simulink model "mBraccioHW"  (R2021a)
settings: Solver=FixedStepAuto  StartTime=0.0  StopTime=inf  RelTol=1e-3  EnableMultiTasking=on
InitFcn:
  | % oJointBase      = classes.Joint(deg2rad(0)-pi/2, deg2rad(180)-pi/2);
  | % oJointShoulder  = classes.Joint(deg2rad(15)-pi/2, deg2rad(165)-pi/2);
  | % oJointElbow     = classes.Joint(deg2rad(0)-pi/2, deg2rad(180)-pi/2);
  | % oJointPitch     = classes.Joint(deg2rad(0)-pi/2, deg2rad(180)-pi/2);
  | % oJointWrist     = classes.Joint(deg2rad(0)-pi/2, deg2rad(180)-pi/2);
  | 
  | % oLinkGround     = classes.Link(70);
  | % oLinkArm        = classes.Link(125);
  | % oLinkForearm    = classes.Link(125);
  | % oLinkHand       = classes.Link(185);
undefined symbols (not defined in the file): adHome, adWS
libraries: arduinolib x13
settings Model: SILPILModeSetting=veronly  ExtModeTrigDuration=2  Creator=angelo  LastModifiedBy=angelo
settings OptimizationCC: EnhancedBackFolding=on  PassReuseOutputArgsAs=Individual arguments  ZeroExternalMemoryAtStartup=off  ZeroInternalMemoryAtStartup=off  MaxStackSize=64  OptimizeBlockOrder=speed  DifferentSizesBufferReuse=on  OptimizationCustomize=off  EfficientTunableParamExpr=on
settings DebuggingCC: ParameterTunabilityLossMsg=error
settings HardwareCC: ProdBitPerInt=16  ProdBitPerPointer=16  ProdBitPerSizeT=16  ProdBitPerPtrDiffT=16  ProdLargestAtomicFloat=None  ProdWordSize=8  ProdHWDeviceType=Atmel->AVR
settings SFSimCC: MATLABDynamicMemAlloc=off
settings RTWCC: SystemTargetFile=ert.tlc  HardwareBoard=Arduino Mega 2560  TemplateMakefile=ert_default_tmf  Toolchain=Arduino AVR  BuildConfiguration=Faster Runs
settings CodeAppCC: ForceParamTrailComments=on  IgnoreCustomStorageClasses=off  OperatorAnnotations=on  SimulinkDataObjDesc=on  SFDataObjDesc=on  InsertBlockDesc=on
settings ERTTargetCC: SupportContinuousTime=on  SupportVariableSizeSignals=on  ExtModeStaticAllocSize=2048

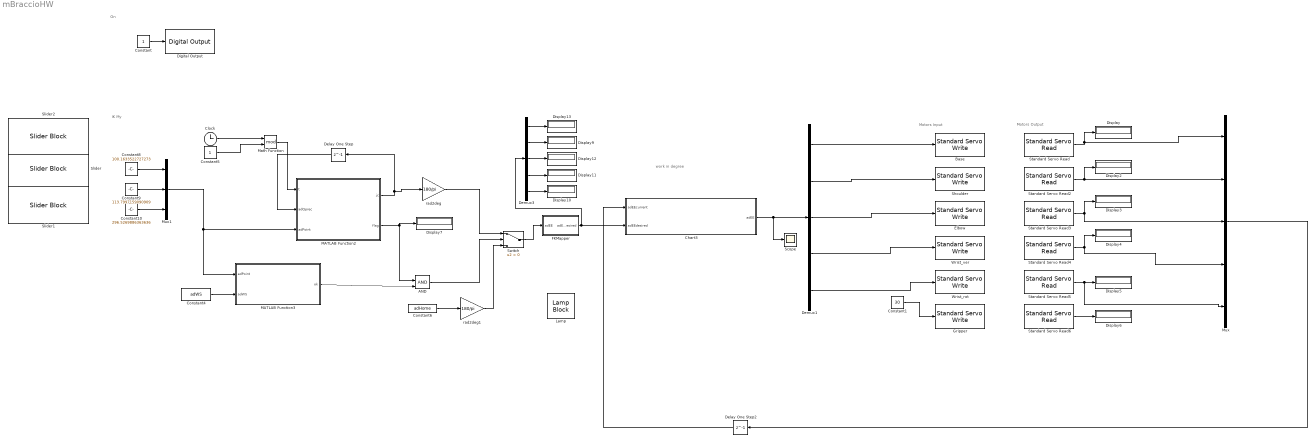
== system mBraccioHW ==
  note: On
  note: IK My
  note: work in degree
  note: Motors Input
  note: Motors Output
  AND : Logic  IconShape=distinctive  AllPortsSameDT=off  OutDataTypeStr=boolean
  Base : arduinolib/Standard Servo Write  pinNumber=11  ServoIndex=0  blockPlatform=ARDUINO
  Chart3 : Stateflow chart  TreatAsAtomicUnit=on  SystemSampleTime=0.02
  Clock : Clock
  Constant : Constant
  Constant1 : Constant  Value=30
  Constant10 : Constant  Value=296.5269886363636
  Constant4 : Constant  Value=adWS
  Constant5 : Constant
  Constant6 : Constant  Value=adHome
  Constant8 : Constant  Value=100.1633522727273
  Constant9 : Constant  Value=113.7997159090909
  Delay One Step : Delay  DelayLength=1  InitialCondition=adHome  SampleTime=0.02
  Delay One Step2 : Delay  DelayLength=1  InitialCondition=[90; 90; 90; 90; 0]
  Demux1 : Demux  Outputs=5
  Demux3 : Demux  Outputs=5
  Digital Output : arduinolib/Digital Output  pinNumber=12  Direction=output  blockPlatform=arduino
  Display{,2..7,9..13} (12 alike) : Display
  Elbow : arduinolib/Standard Servo Write  pinNumber=9  ServoIndex=1  blockPlatform=ARDUINO
  FKMapper : Subsystem
  Gripper : arduinolib/Standard Servo Write  pinNumber=3  ServoIndex=2  blockPlatform=ARDUINO
  Lamp : LampBlock  LabelPosition=Hide
  MATLAB Function2 : MATLAB Function  TreatAsAtomicUnit=on  SystemSampleTime=0.02
  MATLAB Function3 : MATLAB Function  TreatAsAtomicUnit=on  SystemSampleTime=0.02
  Math Function : Math  Operator=mod  SaturateOnIntegerOverflow=on
  Mux : Mux  Inputs=5
  Mux1 : Mux  Inputs=3
  Scope : Scope
  Shoulder : arduinolib/Standard Servo Write  pinNumber=10  ServoIndex=3  blockPlatform=ARDUINO
  Slider : SliderBlock  LabelPosition=Hide  ScaleMax=300
  Slider1 : SliderBlock  LabelPosition=Hide  ScaleMax=300
  Slider2 : SliderBlock  LabelPosition=Hide  ScaleMax=300
  Standard Servo Read : arduinolib/Standard Servo Read  pinNumber=11  SampleTime=0.02  ServoIndex=0  blockPlatform=ARDUINO
      settings: SourceProductBaseCode=ARDUINO
  Standard Servo Read2 : arduinolib/Standard Servo Read  pinNumber=10  SampleTime=0.02  ServoIndex=3  blockPlatform=ARDUINO
      settings: SourceProductBaseCode=ARDUINO
  Standard Servo Read3 : arduinolib/Standard Servo Read  pinNumber=9  SampleTime=0.02  ServoIndex=1  blockPlatform=ARDUINO
      settings: SourceProductBaseCode=ARDUINO
  Standard Servo Read4 : arduinolib/Standard Servo Read  pinNumber=6  SampleTime=0.02  ServoIndex=4  blockPlatform=ARDUINO
      settings: SourceProductBaseCode=ARDUINO
  Standard Servo Read5 : arduinolib/Standard Servo Read  pinNumber=5  SampleTime=0.02  ServoIndex=5  blockPlatform=ARDUINO
      settings: SourceProductBaseCode=ARDUINO
  Standard Servo Read6 : arduinolib/Standard Servo Read  pinNumber=3  SampleTime=0.02  ServoIndex=2  blockPlatform=ARDUINO
      settings: SourceProductBaseCode=ARDUINO
  Switch : Switch  Criteria=u2 > Threshold
  Wrist_rot : arduinolib/Standard Servo Write  pinNumber=5  ServoIndex=5  blockPlatform=ARDUINO
  Wrist_ver : arduinolib/Standard Servo Write  pinNumber=6  ServoIndex=4  blockPlatform=ARDUINO
  rad2deg : Gain  Gain=180/pi
  rad2deg1 : Gain  Gain=180/pi
  wires:
  Constant/1 -> Digital Output/1
  Demux3/1 -> Display13/1
  Demux3/3 -> Display12/1
  Demux3/5 -> Display10/1
  Demux3/2 -> Display9/1
  Demux3/4 -> Display11/1
  Chart3/1(adEE) -> Scope/1, Demux1/1
  Standard Servo Read3/1 -> Display3/1, Mux/3
  Standard Servo Read4/1 -> Display4/1, Mux/4
  Standard Servo Read6/1 -> Display6/1
  Standard Servo Read2/1 -> Display2/1, Mux/2
  Standard Servo Read/1 -> Display/1, Mux/1
  Standard Servo Read5/1 -> Display5/1, Mux/5
  Delay One Step2/1 -> Chart3/1(adEEcurrent)
  Demux1/1 -> Base/1
  Demux1/2 -> Shoulder/1
  Demux1/3 -> Elbow/1
  Demux1/4 -> Wrist_ver/1
  Demux1/5 -> Wrist_rot/1
  Constant1/1 -> Gripper/1
  MATLAB Function2/2(flag) -> Display7/1, AND/1
  Constant8/1 -> Mux1/1
  Constant9/1 -> Mux1/2
  Constant10/1 -> Mux1/3
  Mux1/1 -> MATLAB Function3/1(adPoint), MATLAB Function2/3(adPoint)
  MATLAB Function2/1(jc) -> Delay One Step/1, rad2deg/1
  Constant4/1 -> MATLAB Function3/2(adWS)
  MATLAB Function3/1(ok) -> AND/2
  Switch/1 -> FKMapper/1(adEE)
  AND/1 -> Switch/2
  rad2deg/1 -> Switch/1
  Constant6/1 -> rad2deg1/1
  rad2deg1/1 -> Switch/3
  Mux/1 -> Delay One Step2/1
  FKMapper/1(adEEdesired) -> Chart3/2(adEEdesired), Demux3/1
  Clock/1 -> Math Function/1
  Constant5/1 -> Math Function/2
  Math Function/1 -> MATLAB Function2/1(t)
  Delay One Step/1 -> MATLAB Function2/2(adQprec)

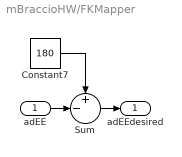
== system mBraccioHW/FKMapper ==
  adEE : Inport
  Constant7 : Constant  Value=180
  Sum : Sum  Inputs=+-|
  adEEdesired : Outport
  wires:
  Sum/1 -> adEEdesired/1
  adEE/1 -> Sum/2
  Constant7/1 -> Sum/1

== matlab function mBraccioHW/MATLAB Function2 ==
  data: t input; adQprec input; adPoint input; jc output; flag output
function [jc, flag] = ikin(t, adQprec, adPoint)
if(t ~= 0)
    flag  	= true;
    jc      = adQprec;
    return;
end

% Joints definition
oJointBase      = classes.Joint(deg2rad(0)-pi/2, deg2rad(180)-pi/2);
oJointShoulder  = classes.Joint(deg2rad(15)-pi/2, deg2rad(165)-pi/2);
oJointElbow     = classes.Joint(deg2rad(0)-pi/2, deg2rad(180)-pi/2);
oJointPitch     = classes.Joint(deg2rad(0)-pi/2, deg2rad(180)-pi/2);
oJointWrist     = classes.Joint(deg2rad(0)-pi/2, deg2rad(180)-pi/2);

% Liks definition
oLinkGround     = classes.Link(70);
oLinkArm        = classes.Link(125);
oLinkForearm    = classes.Link(125);
oLinkHand       = classes.Link(185);

% Braccio definition
oBraccio        = classes.Robot5Dof(oJointBase, oJointShoulder,     ...
                                    oJointElbow, oJointPitch,       ... 
                                    oJointWrist, oLinkGround,       ...
                                    oLinkArm, oLinkForearm,         ...
                                    oLinkHand);

% IKIN computation
[bOK, adQ]      = oBraccio.IKIN(adPoint);
adQ(1)          = adQ(1)-pi/2;

% Output
jc              = [adQ+pi/2; 0];
flag            = bOK;
end

== stateflow chart mBraccioHW/Chart3 ==
  settings: executeAtInitialization=1
  state First
    during:
    adEE = [
    nextStep(adEEcurrent(1), adEEdesired(1));
    nextStep(adEEcurrent(2), adEEdesired(2));
    nextStep(adEEcurrent(3), adEEdesired(3));
    nextStep(adEEcurrent(4), adEEdesired(4));
    nextStep(adEEcurrent(5), adEEdesired(5)) ];
  (default) -> First
  data: current function_input; desired function_input; v function_output; adEEcurrent input; adEE output; adEEdesired input
  function v = nextStep(current, desired):
    | function v = nextStep(current, desired)
    | if (current < desired)
    |     current = current + 1;
    | end
    | 
    | if (current > desired)
    |     current = current - 1;
    | end
    | 
    | v = current;
    | end

== matlab function mBraccioHW/MATLAB Function3 ==
  data: adPoint input; ok output; adWS input
function ok = verifierWS(adPoint, adWS)
ok = functions.isInsideWorkspace(adPoint, adWS(1), adWS(2), adWS(3));
end
